simulink model "kalman_filter"  (R2015b)
settings: Solver=VariableStepAuto  StartTime=0.0  StopTime=10.0  RelTol=1e-3
values from neighbouring files (symbols this model uses):
  A = [1,2,3 ... (first row only)    [jacobian_test.m]
undefined symbols (not defined in the file or in its folder): g, KetaD, KetaP, KF_P0, KF_Q, KF_R, m
settings Model: Creator=mgreiff  LastModifiedBy=mgreiff

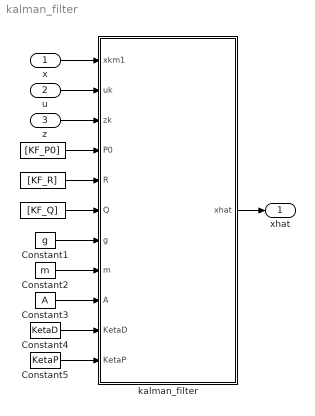
== system kalman_filter ==
  x : Inport  PortDimensions=10
  u : Inport  Port=2  PortDimensions=3
  z : Inport  Port=3  PortDimensions=6
  " " : Constant  Value=[KF_P0]
  "  " : Constant  Value=[KF_R]
  "   " : Constant  Value=[KF_Q]
  Constant1 : Constant  Value=g
  Constant2 : Constant  Value=m
  Constant3 : Constant  Value=A
  Constant4 : Constant  Value=KetaD
  Constant5 : Constant  Value=KetaP
  kalman_filter : MATLAB Function  TreatAsAtomicUnit=on
  xhat : Outport  PortDimensions=10
  wires:
  x/1 -> kalman_filter/1(xkm1)
  u/1 -> kalman_filter/2(uk)
  z/1 -> kalman_filter/3(zk)
  " "/1 -> kalman_filter/4(P0)
  "  "/1 -> kalman_filter/5(R)
  "   "/1 -> kalman_filter/6(Q)
  kalman_filter/1(xhat) -> xhat/1
  Constant3/1 -> kalman_filter/9(A)
  Constant2/1 -> kalman_filter/8(m)
  Constant1/1 -> kalman_filter/7(g)
  Constant4/1 -> kalman_filter/10(KetaD)
  Constant5/1 -> kalman_filter/11(KetaP)

== matlab function kalman_filter/kalman_filter ==
  data: xhat output; xkm1 input; uk input; zk input; P0 input; R input; Q input; g input; m input; A input; KetaD input; KetaP input
function xhat  = fcn(xkm1, uk, zk, P0, R, Q, g, m, A, KetaD, KetaP)
%#codegen
% xkm1  = [x,             uk = [e_z,         zk = [z,
%          y,                   e_phi,             dotx,
%          z,                   e_theta]           doty,
%          dotx,                                   dotz,
%          doty,                                   theta,
%          dotz,                                   phi]
%          phi,
%          theta,
%          dotphi,
%          dottheta]

persistent P

if isempty(P)
    P = P0;
end
%% Set up basic continuous-model dynamics, including PD
Ad = diag(A);
a1 = 4.8; a2 = 8.32; b = 8.32;
a1 = KetaD(1); a2 = KetaP(1); b = KetaP(1);

T0 = m*g;

A1 = zeros(10,3);
A2 = [eye(3); -Ad/m; zeros(4,3)];
A3 = [zeros(3,2); T0/m, 0; 0, -T0/m; zeros(3,2); -a2*eye(2)];
A4 = [zeros(6,2); eye(2); -a1*eye(2)];
Ac = [A1,A2,A3,A4];

Bc = zeros(10, 3);
Bc(6, 1) = 1/m;
Bc(9, 2) = b;
Bc(10, 3) = b;

Cc = zeros(6, 10);
Cc(1,3) = 1;
Cc(2:6,4:8) = eye(5);

Dc = zeros(6, 3);

%[Ad, Bd, Cd, Dd] = ssdata(c2d(ss(Ac,Bc,Cc,Dc),0.01));

% Predictor step
xf = Ac * xkm1 + Bc * uk;
Pf = Ac * P * Ac' + Q;

% Corrector step
K =  Pf * Cc' / (Cc * Pf * Cc'+ R);
xhat = xf + K * (zk - Cc * xf);
P = (eye(10) - K * Cc) * Pf;
